simulink model "ACC_Model_frontspeedout1"  (Simulink 7.9)
settings: Solver=ode5  StartTime=0.0  StopTime=200  FixedStep=0.2  RelTol=1e-3
undefined symbols (not defined in the file): sigbuilder_block
libraries: simulink x1
settings Model: Creator=kamesh  LastModifiedBy=Neel
settings DataIOCC: FinalStateName=SimState  LimitDataPoints=off  MaxDataPoints=10  SaveCompleteFinalSimState=on
settings OptimizationCC: InlineParams=on  UseFloatMulNetSlope=on  UseSpecifiedMinMax=on  InlineInvariantSignals=on  EnhancedBackFolding=on  ZeroExternalMemoryAtStartup=off  ZeroInternalMemoryAtStartup=off  NoFixptDivByZeroProtection=on  EfficientFloat2IntCast=on  OptimizeModelRefInitCode=on  LifeSpan=1
settings DebuggingCC: SolverPrmCheckMsg=none
settings HardwareCC: ProdBitPerInt=16  ProdBitPerPointer=16  ProdIntDivRoundTo=Floor  ProdEndianess=BigEndian  ProdWordSize=16  ProdHWDeviceType=Freescale->HC(S)12
settings RTWCC: SystemTargetFile=ert.tlc  GenCodeOnly=on  TemplateMakefile=ert_default_tmf  PostCodeGenCommand=packNGo(buildInfo, {'packType' 'hierarchical'})  Description=Embedded Coder  GenerateReport=on  ProcessScript=ert_make_rtw_hook  IncludeHyperlinkInReport=on  LaunchReport=on  GenerateCodeMetricsReport=on  RTWCompilerOptimization=On
settings CodeAppCC: IgnoreCustomStorageClasses=off  MATLABSourceComments=on
settings ERTTargetCC: CodeReplacementLibrary=ANSI_C  MultiwordLength=2048  GenerateSampleERTMain=on  InlinedParameterPlacement=NonHierarchical  ERTCustomFileTemplate=example_file_process.tlc  ConvertIfToSwitch=off  SuppressUnreachableDefaultCases=off

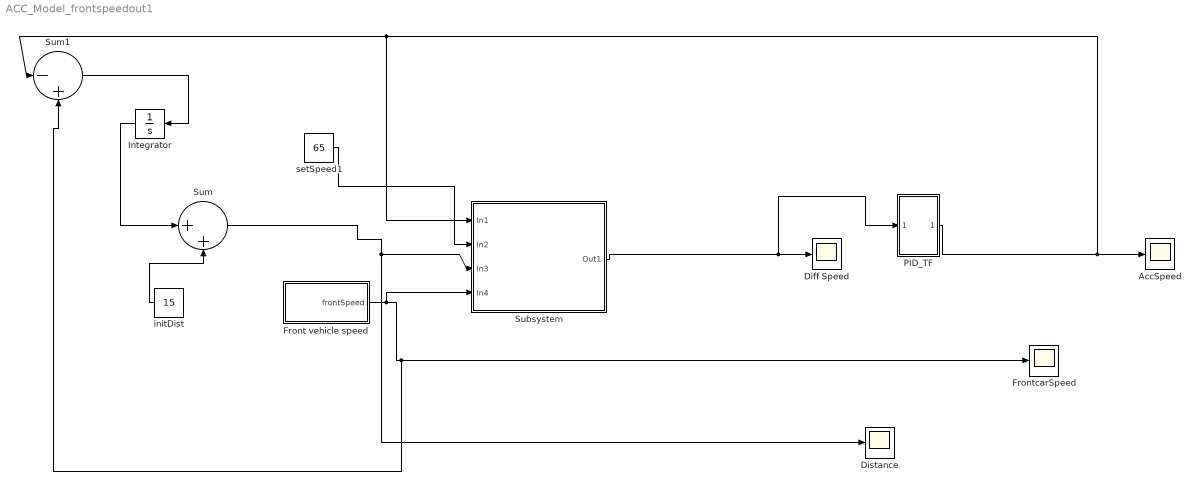
== system ACC_Model_frontspeedout1 ==
  AccSpeed : Scope
  Diff Speed : Scope
  Distance : Scope
      settings: SaveName=ScopeData2
  Front vehicle speed : Subsystem  Tag=STV Subsys  LoadFcn=sigbuilder_block('load');  StartFcn=sigbuilder_block('start');  StopFcn=sigbuilder_block('stop');  ClipboardFcn=sigbuilder_block('clipboard');  mask(Sigbuilder block){}
      mask help: Simulink:masks:SigbuilderBlock_MD
      mask init:
      | if ~strcmp(get_param(bdroot(gcbh),'SimulationStatus'),'stopped') tuvar = sigbuilder_block('maskInit'); end
      settings: CopyFcn=sigbuilder_block('copy');  DeleteFcn=sigbuilder_block('delete');  ModelCloseFcn=sigbuilder_block('modelClose');  PreSaveFcn=sigbuilder_block('preSave');  PauseFcn=sigbuilder_block('pause');  ContinueFcn=sigbuilder_block('continue');  NameChangeFcn=sigbuilder_block('namechange');  OpenFcn=sigbuilder_block('open',[410.25 112.5 550.5 394.5 ]);  CloseFcn=sigbuilder_block('close');
      mask Display: plot(0, 0, 100, 100,[2, 2, 32, 32, 2], [68, 8, 8, 68, 68],[32, 2], [38, 38], [32, 19, 2],[53, 60, 44], [32, 17, 17, 2],[16, 16, 31, 31]);txt = getActiveGroup(gcbh);text(2, 100, txt,'verticalAlignment', 'top');
  FrontcarSpeed : Scope
      settings: TimeRange=200  SaveName=ScopeData3
  Integrator : Integrator
  PID_TF : Subsystem
  Subsystem : Subsystem
  Sum : Sum  Inputs=|++
  Sum1 : Sum  Inputs=|-+
  initDist : Constant  Value=15
  setSpeed1 : Constant  Value=65
  wires:
  PID_TF/1(Out1) -> AccSpeed/1, Sum1/1, Subsystem/1(In1)
  initDist/1 -> Sum/2
  Subsystem/1(Out1) -> Diff Speed/1, PID_TF/1(In1)
  Sum/1 -> Subsystem/3(In3), Distance/1
  Front vehicle speed/1(frontSpeed) -> Subsystem/4(In4), Sum1/2, FrontcarSpeed/1
  setSpeed1/1 -> Subsystem/2(In2)
  Sum1/1 -> Integrator/1
  Integrator/1 -> Sum/1

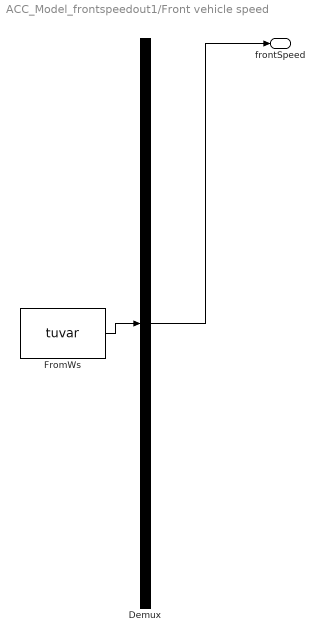
== system ACC_Model_frontspeedout1/Front vehicle speed ==
  Demux : Demux  Tag=STV Demux  Outputs=1
  FromWs : FromWorkspace  Tag=STV FromWs  VariableName=tuvar  SampleTime=0  SigBuilderData=DataTag0  VnvData=DataTag1
      SigBuilderData=|
      | common.afterFinalStr = 'Extrapolate'
      | common.sampleTime = 0
      | dataSet.timeRange = [0 200]
      | dataSet.name = 'Group 1'
      | sbobj.Groups.Name = 'Group 1'
      | sbobj.Groups.Signals.Name = 'frontSpeed'
      | sbobj.Groups.Signals.XData = [0 18 25 45 80 200]
      | sbobj.Groups.Signals.YData = [62 25 25 30 35.05 69.8]
      | sbobj.Groups.TimeRange = [0 200]
  frontSpeed : Outport  Tag=STV Outport
  wires:
  Demux/1 -> frontSpeed/1
  FromWs/1 -> Demux/1

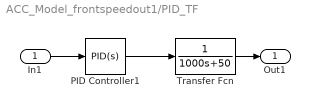
== system ACC_Model_frontspeedout1/PID_TF ==
  In1 : Inport
  PID Controller1 : simulink/Continuous/PID Controller  Controller=PID  TimeDomain=Continuous-time  SampleTime=1  IntegratorMethod=Forward Euler  FilterMethod=Forward Euler  Form=Parallel  P=2000  I=80  D=0  N=100  InitialConditionSource=internal  InitialConditionForIntegrator=0  InitialConditionForFilter=0  ExternalReset=none  LimitOutput=off  UpperSaturationLimit=inf  LowerSaturationLimit=-inf  LinearizeAsGain=off  AntiWindupMode=none  Kb=1  TrackingMode=off  Kt=1  PParamMin=[]  PParamMax=[]  IParamMin=[]  IParamMax=[]  DParamMin=[]  DParamMax=[]  NParamMin=[]  NParamMax=[]  KbParamMin=[]  KbParamMax=[]  KtParamMin=[]  KtParamMax=[]  POutMin=[]  POutMax=[]  IOutMin=[]  IOutMax=[]  DOutMin=[]  DOutMax=[]  NOutMin=[]  NOutMax=[]  KbOutMin=[]  KbOutMax=[]  KtOutMin=[]  KtOutMax=[]  IntegratorOutMin=[]  IntegratorOutMax=[]  FilterOutMin=[]  FilterOutMax=[]  SumOutMin=[]  SumOutMax=[]  SumI1OutMin=[]  SumI1OutMax=[]  SumI2OutMin=[]  SumI2OutMax=[]  SumI3OutMin=[]  SumI3OutMax=[]  SumDOutMin=[]  SumDOutMax=[]  SaturationOutMin=[]  SaturationOutMax=[]  IntegratorContinuousStateAttributes=''  IntegratorStateMustResolveToSignalObject=off  IntegratorRTWStateStorageClass=Auto  FilterContinuousStateAttributes=''  FilterStateMustResolveToSignalObject=off  FilterRTWStateStorageClass=Auto
  Transfer Fcn : TransferFcn  Denominator=[1000 50]
  Out1 : Outport
  wires:
  PID Controller1/1 -> Transfer Fcn/1
  In1/1 -> PID Controller1/1
  Transfer Fcn/1 -> Out1/1

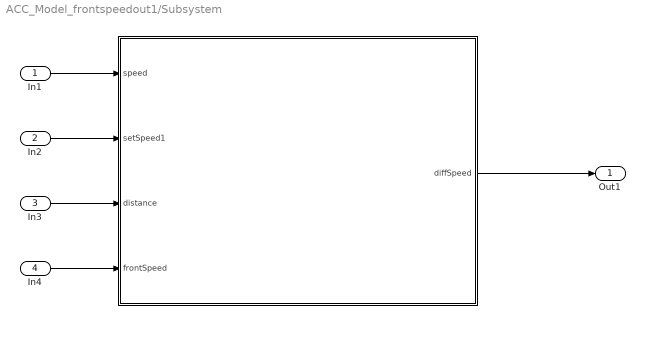
== system ACC_Model_frontspeedout1/Subsystem ==
  In1 : Inport
  In2 : Inport  Port=2
  In3 : Inport  Port=3
  In4 : Inport  Port=4
  "          " : MATLAB Function  TreatAsAtomicUnit=on
  Out1 : Outport
  wires:
  In3/1 -> "          "/3(distance)
  "          "/1(diffSpeed) -> Out1/1
  In4/1 -> "          "/4(frontSpeed)
  In2/1 -> "          "/2(setSpeed1)
  In1/1 -> "          "/1(speed)

== matlab function Subsystem/           ==
  data: speed input double; setSpeed1 input double; diffSpeed output double; distance input double; frontSpeed input double
function diffSpeed  = AccSubsystem(speed,setSpeed1,distance,frontSpeed)
timeC=0.2;
acc_C = 8.5;
des_distance=30;
persistent setSpeed;
if isempty(setSpeed)
    setSpeed= 0;
end

minSpeed = 10;

deltaX=((frontSpeed*frontSpeed)-(speed*speed))/(2*(-acc_C));


if(distance<=(des_distance + (deltaX)))
    if(distance <= deltaX + des_distance) && (distance  >= des_distance)
        
        tmpSpeed1 = sqrt((speed * speed) + (2*(-acc_C)*abs((deltaX + des_distance)-distance)));
        setSpeed = max(frontSpeed,tmpSpeed1);      % stops the reduction at front_speed.
        
        
    elseif(distance <des_distance)
        tmpSpeed2 = sqrt((speed * speed) + (2*(-acc_C)*abs(des_distance-distance)));
        setSpeed = max(minSpeed,tmpSpeed2);
        
    end
elseif(distance>(des_distance + (deltaX)))
    setSpeed = speed + (acc_C*timeC);% v = u + at
    %setSpeed = min(setSpeed1,tmpSpeed3);
    
end
 setSpeed = min(setSpeed1,setSpeed);
diffSpeed = setSpeed - speed;


end
